simulink model "dz_5"  (R2022b)
settings: Solver=FixedStepAuto  StartTime=0.0  StopTime=30  FixedStep=0.001  RelTol=1e-3
settings Model: Creator=osini  LastModifiedBy=osini

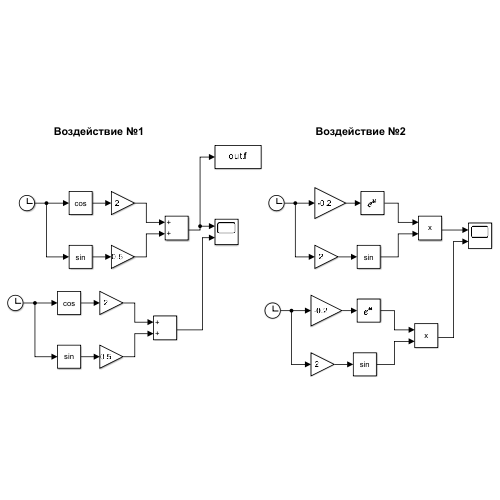
[thumbnail: Simulink's stored preview of the top-level diagram]
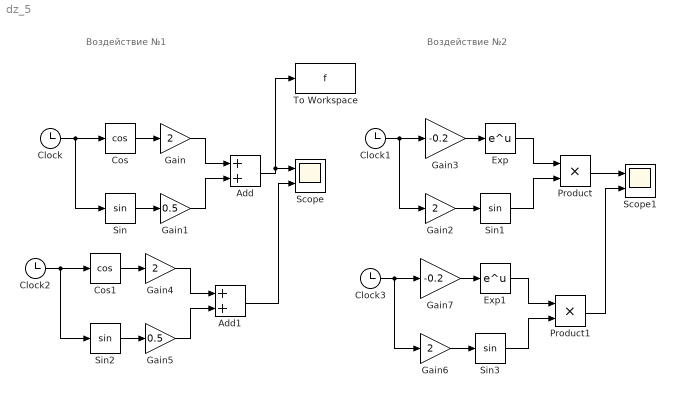
== system dz_5 ==
  note: Воздействие №1
  note: Воздействие №2
  Add : Sum
  Add1 : Sum
  Clock{,1..3} (4 alike) : Clock
  Cos : Trigonometry  Operator=cos
  Cos1 : Trigonometry  Operator=cos
  Exp : Math
  Exp1 : Math
  Gain{,2,4,6} (4 alike) : Gain  Gain=2
  Gain1 : Gain  Gain=0.5
  Gain3 : Gain  Gain=-0.2
  Gain5 : Gain  Gain=0.5
  Gain7 : Gain  Gain=-0.2
  Product : Product
  Product1 : Product
  Scope : Scope  NumInputPorts=2
  Scope1 : Scope  NumInputPorts=2
  Sin{,1..3} (4 alike) : Trigonometry
  To Workspace : ToWorkspace  VariableName=f  SaveFormat=Structure With Time  SampleTime=0.001
  wires:
  Clock/1 -> Sin/1, Cos/1
  Cos/1 -> Gain/1
  Sin/1 -> Gain1/1
  Gain/1 -> Add/1
  Gain1/1 -> Add/2
  Add/1 -> To Workspace/1, Scope/1
  Gain2/1 -> Sin1/1
  Clock1/1 -> Gain2/1, Gain3/1
  Gain3/1 -> Exp/1
  Exp/1 -> Product/1
  Sin1/1 -> Product/2
  Product/1 -> Scope1/1
  Cos1/1 -> Gain4/1
  Sin2/1 -> Gain5/1
  Clock2/1 -> Sin2/1, Cos1/1
  Add1/1 -> Scope/2
  Gain5/1 -> Add1/2
  Gain4/1 -> Add1/1
  Exp1/1 -> Product1/1
  Gain6/1 -> Sin3/1
  Sin3/1 -> Product1/2
  Clock3/1 -> Gain6/1, Gain7/1
  Gain7/1 -> Exp1/1
  Product1/1 -> Scope1/2
